simulink model "tri5"  (R2016b)
settings: Solver=VariableStepAuto  StartTime=0.0  StopTime=20  RelTol=1e-3
settings Model: Creator=Admin  LastModifiedBy=Admin

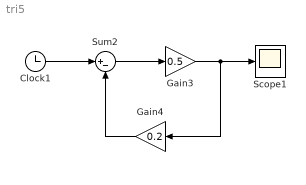
== system tri5 ==
  Clock1 : Clock
  Gain3 : Gain  Gain=0.5
  Gain4 : Gain  Gain=0.2
  Scope1 : Scope
  Sum2 : Sum  Inputs=|+-
  wires:
  Clock1/1 -> Sum2/1
  Sum2/1 -> Gain3/1
  Gain3/1 -> Gain4/1, Scope1/1
  Gain4/1 -> Sum2/2
